simulink subsystem "Plant"  (R2024b)
settings: Solver=VariableStepAuto  StartTime=0.0  StopTime=10.0  RelTol=1e-3
values from neighbouring files (symbols this model uses):
  actuator_delay = 0.1131    [TADPOLEControl.m]
  ipaError = consts(6)    [NonLinearModel.m]
  oxDensityArray = fuelData(1,:)    [MDotODE.m]    (also in oxangle2mdot.m)
  oxError = consts(5)    [NonLinearModel.m]
  oxPressureArray = fuelData(2,:)    [MDotODE.m]    (also in oxangle2mdot.m)
  PcError = consts(7)    [NonLinearModel.m]
undefined symbols (not defined in the file or in its folder): consts, simData, thrustArray
libraries: dspobslib x5
settings Model: Creator=rober  LastModifiedBy=pplat

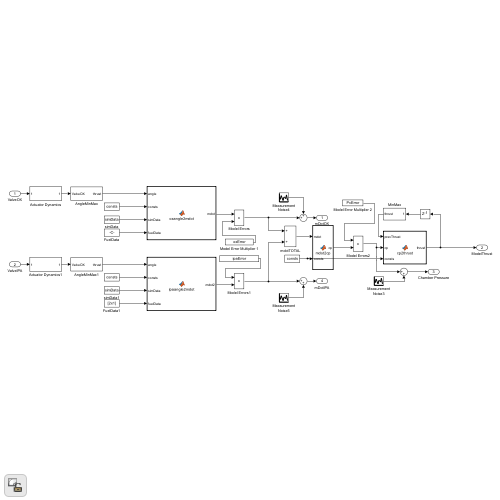
[thumbnail: Simulink's stored preview of the top-level diagram]
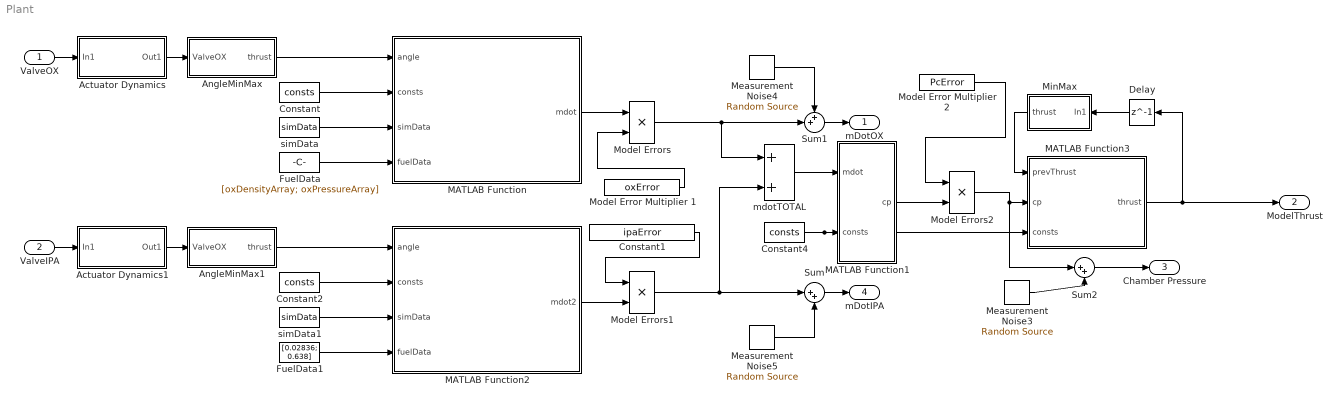
== system Plant ==
  ValveOX : Inport
  ValveIPA : Inport  Port=2
  Actuator Dynamics : Subsystem
  Actuator Dynamics1 : Subsystem
  AngleMinMax : Subsystem
  AngleMinMax1 : Subsystem
  Constant : Constant  Value=consts
  Constant1 : Constant  Value=ipaError
  Constant2 : Constant  Value=consts
  Constant4 : Constant  Value=consts
  Delay : Delay  DelayLength=1  InitialCondition=0  InputProcessing=Columns as channels (frame based)
  FuelData : Constant  Value=[oxDensityArray; oxPressureArray]
  FuelData1 : Constant  Value=[0.02836; 0.638]
  MATLAB Function : MATLAB Function  TreatAsAtomicUnit=on
  MATLAB Function1 : MATLAB Function  TreatAsAtomicUnit=on
  MATLAB Function2 : MATLAB Function  TreatAsAtomicUnit=on
  MATLAB Function3 : MATLAB Function  TreatAsAtomicUnit=on
  Measurement Noise3 : dspobslib/Random Source  SrcType=Gaussian  NormMethod=Ziggurat  CltLength=12  MinVal=0  MaxVal=1  MeanVal=0  VarVal=noise_var_outputs  RepMode=Not repeatable  rawSeed=1  IsInherit=off  SampMode=Continuous  SampTime=1  SampFrame=1  DataType=Double  OutComplex=Real  OutputFrames=off
  Measurement Noise4 : dspobslib/Random Source  SrcType=Gaussian  NormMethod=Ziggurat  CltLength=12  MinVal=0  MaxVal=1  MeanVal=0  VarVal=noise_var_mdot  RepMode=Not repeatable  rawSeed=1  IsInherit=off  SampMode=Continuous  SampTime=1  SampFrame=1  DataType=Double  OutComplex=Real  OutputFrames=off
  Measurement Noise5 : dspobslib/Random Source  SrcType=Gaussian  NormMethod=Ziggurat  CltLength=12  MinVal=0  MaxVal=1  MeanVal=0  VarVal=noise_var_mdot  RepMode=Not repeatable  rawSeed=1  IsInherit=off  SampMode=Continuous  SampTime=1  SampFrame=1  DataType=Double  OutComplex=Real  OutputFrames=off
  MinMax : Subsystem
  Model Error Multiplier 1 : Constant  Value=oxError
  Model Error Multiplier 2 : Constant  Value=PcError
  Model Errors : Product
  Model Errors1 : Product
  Model Errors2 : Product
  Sum : Sum  Inputs=|++
  Sum1 : Sum  Inputs=++|
  Sum2 : Sum  Inputs=|++
  mdotTOTAL : Sum
  simData : Constant  Value=simData
  simData1 : Constant  Value=simData
  mDotOX : Outport
  ModelThrust : Outport  Port=2
  Chamber Pressure : Outport  Port=3
  mDotIPA : Outport  Port=4
  wires:
  Constant/1 -> MATLAB Function/2(consts)
  FuelData/1 -> MATLAB Function/4(fuelData)
  FuelData1/1 -> MATLAB Function2/4(fuelData)
  Constant2/1 -> MATLAB Function2/2(consts)
  Constant4/1 -> MATLAB Function1/2(consts), MATLAB Function3/3(consts)
  mdotTOTAL/1 -> MATLAB Function1/1(mdot)
  Delay/1 -> MinMax/1(In1)
  MinMax/1(thrust) -> MATLAB Function3/1(prevThrust)
  simData/1 -> MATLAB Function/3(simData)
  simData1/1 -> MATLAB Function2/3(simData)
  MATLAB Function3/1(thrust) -> Delay/1, ModelThrust/1
  ValveOX/1 -> Actuator Dynamics/1(In1)
  Actuator Dynamics/1(Out1) -> AngleMinMax/1(ValveOX)
  ValveIPA/1 -> Actuator Dynamics1/1(In1)
  Actuator Dynamics1/1(Out1) -> AngleMinMax1/1(ValveOX)
  Sum/1 -> mDotIPA/1
  Measurement Noise5/1 -> Sum/2
  Sum1/1 -> mDotOX/1
  Measurement Noise3/1 -> Sum2/2
  Sum2/1 -> Chamber Pressure/1
  Model Errors/1 -> mdotTOTAL/1, Sum1/2
  MATLAB Function/1(mdot) -> Model Errors/1
  MATLAB Function2/1(mdot2) -> Model Errors1/2
  Model Errors1/1 -> Sum/1, mdotTOTAL/2
  Model Error Multiplier 1/1 -> Model Errors/2
  AngleMinMax/1(thrust) -> MATLAB Function/1(angle)
  AngleMinMax1/1(thrust) -> MATLAB Function2/1(angle)
  Constant1/1 -> Model Errors1/1
  Model Errors2/1 -> Sum2/1, MATLAB Function3/2(cp)
  MATLAB Function1/1(cp) -> Model Errors2/2
  Model Error Multiplier 2/1 -> Model Errors2/1
  Measurement Noise4/1 -> Sum1/1

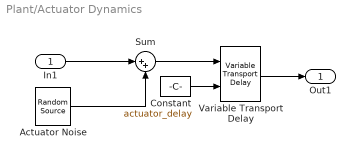
== system Plant/Actuator Dynamics ==
  In1 : Inport
  Actuator Noise : dspobslib/Random Source  SrcType=Gaussian  NormMethod=Ziggurat  CltLength=12  MinVal=0  MaxVal=1  MeanVal=0  VarVal=noise_var_actuators  RepMode=Not repeatable  rawSeed=1  IsInherit=off  SampMode=Continuous  SampTime=1  SampFrame=1  DataType=Double  OutComplex=Real  OutputFrames=off
  Constant : Constant  Value=actuator_delay
  Sum : Sum  Inputs=|++
  Variable Transport Delay : VariableTransportDelay  VariableDelayType=Variable transport delay  MaximumDelay=10  InitialOutput=50  MaximumPoints=2048
  Out1 : Outport
  wires:
  Sum/1 -> Variable Transport Delay/1
  Variable Transport Delay/1 -> Out1/1
  Constant/1 -> Variable Transport Delay/2
  In1/1 -> Sum/1
  Actuator Noise/1 -> Sum/2

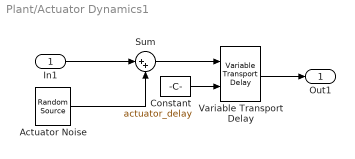
== system Plant/Actuator Dynamics1 ==
  In1 : Inport
  Actuator Noise : dspobslib/Random Source  SrcType=Gaussian  NormMethod=Ziggurat  CltLength=12  MinVal=0  MaxVal=1  MeanVal=0  VarVal=noise_var_actuators  RepMode=Not repeatable  rawSeed=1  IsInherit=off  SampMode=Continuous  SampTime=1  SampFrame=1  DataType=Double  OutComplex=Real  OutputFrames=off
  Constant : Constant  Value=actuator_delay
  Sum : Sum  Inputs=|++
  Variable Transport Delay : VariableTransportDelay  VariableDelayType=Variable transport delay  MaximumDelay=10  InitialOutput=60  MaximumPoints=2048
  Out1 : Outport
  wires:
  Sum/1 -> Variable Transport Delay/1
  Variable Transport Delay/1 -> Out1/1
  Constant/1 -> Variable Transport Delay/2
  In1/1 -> Sum/1
  Actuator Noise/1 -> Sum/2

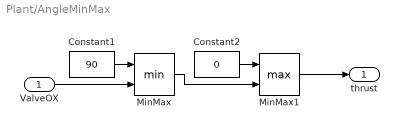
== system Plant/AngleMinMax ==
  ValveOX : Inport
  Constant1 : Constant  Value=90
  Constant2 : Constant  Value=0
  MinMax : MinMax  Inputs=2
  MinMax1 : MinMax  Function=max  Inputs=2
  thrust : Outport
  wires:
  MinMax1/1 -> thrust/1
  ValveOX/1 -> MinMax/2
  MinMax/1 -> MinMax1/2
  Constant1/1 -> MinMax/1
  Constant2/1 -> MinMax1/1

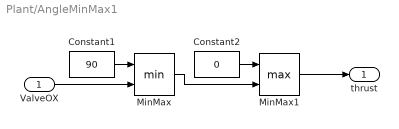
== system Plant/AngleMinMax1 ==
  ValveOX : Inport
  Constant1 : Constant  Value=90
  Constant2 : Constant  Value=0
  MinMax : MinMax  Inputs=2
  MinMax1 : MinMax  Function=max  Inputs=2
  thrust : Outport
  wires:
  MinMax1/1 -> thrust/1
  ValveOX/1 -> MinMax/2
  MinMax/1 -> MinMax1/2
  Constant1/1 -> MinMax/1
  Constant2/1 -> MinMax1/1

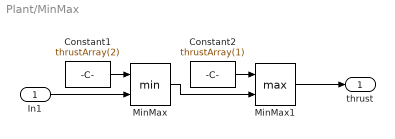
== system Plant/MinMax ==
  In1 : Inport
  Constant1 : Constant  Value=thrustArray(2)
  Constant2 : Constant  Value=thrustArray(1)
  MinMax : MinMax  Inputs=2
  MinMax1 : MinMax  Function=max  Inputs=2
  thrust : Outport
  wires:
  MinMax1/1 -> thrust/1
  In1/1 -> MinMax/2
  MinMax/1 -> MinMax1/2
  Constant1/1 -> MinMax/1
  Constant2/1 -> MinMax1/1

== matlab function Plant/MATLAB Function ==
  data: angle input; mdot output; consts input; simData input; fuelData input
function mdot = oxangle2mdot(angle, consts, simData, fuelData)

    % Conversion Factors and LookUp Arrays
    conversionFactors = [0.004329 60 0.000453592 61023.7];
    subCritVArray = [0.000, 0.070, 0.161, 0.378, 0.670, 1.000, 1.450, 2.050, 2.780, 3.710, 4.960];
    valveAngleArray = [0, 9, 18, 27, 36, 45, 54, 63, 72, 81, 90];
    tempArray = [55, 60, 65, 70, 75, 80, 85, 90, 95, 100, 105, 110, ...
    115, 120, 125, 130, 135, 140, 145, 150];
    oxDensityArray = fuelData(1,:);
    oxPressureArray = fuelData(2,:);

    % cV lookup based off of angle
    subCritV = interp1(valveAngleArray, subCritVArray, angle);

    % ox
    throat = 0.00989;
    cd = 0.975;

    % density and vapour pressure ox
    simData(4);
    density_cv = interp1(tempArray, oxDensityArray, simData(4));
    p_vap = interp1(tempArray, oxPressureArray, simData(4));
    density_valve = interp1(tempArray, oxDensityArray, simData(3));

    %Generates mdot
    alpha = conversionFactors(1)*conversionFactors(2);
    gamma = cd^2*throat^2*2*density_cv*(consts(3)*12);
    beta = conversionFactors(3)*conversionFactors(4);
    deltaP = simData(1)-p_vap;
    mdot = sqrt(subCritV^2*density_valve*(deltaP)*gamma /...
        (alpha^2*gamma*beta + subCritV^2*density_valve));
end

== matlab function Plant/MATLAB Function1 ==
  data: mdot input; cp output; consts input
function cp = mdot2cp(mdot, consts)
    
    cp = mdot*consts(2) / (consts(1)*consts(3));
end

== matlab function Plant/MATLAB Function2 ==
  data: angle input; mdot2 output; consts input; simData input; fuelData input
function mdot2 = ipaangle2mdot(angle, consts, simData, fuelData)

    % Conversion Factors and LookUp Arrays
    conversionFactors = [0.004329 60 0.000453592 61023.7];
    subCritVArray = [0.000, 0.070, 0.161, 0.378, 0.670, 1.000, 1.450, 2.050, 2.780, 3.710, 4.960];
    valveAngleArray = [0, 9, 18, 27, 36, 45, 54, 63, 72, 81, 90];
    tempArray = [55, 60, 65, 70, 75, 80, 85, 90, 95, 100, 105, 110, ...
    115, 120, 125, 130, 135, 140, 145, 150];
    ipaDensityArray = fuelData(1,:);
    ipaPressureArray = fuelData(2,:);

    % cV lookup based off of angle
    subCritV = interp1(valveAngleArray, subCritVArray, angle);

    % ox
    throat = 0.00989;
    cd = 0.975;

    % density and vapour pressure ox
    simData(4);
    density_cv = ipaDensityArray;
    p_vap = ipaPressureArray;
    density_valve = ipaDensityArray;

    %Generates mdot
    alpha = conversionFactors(1)*conversionFactors(2);
    gamma = cd^2*throat^2*2*density_cv*(consts(3)*12);
    beta = conversionFactors(3)*conversionFactors(4);
    deltaP = simData(1)-p_vap;
    mdot2 = sqrt(subCritV^2*density_valve*(deltaP)*gamma /...
        (alpha^2*gamma*beta + subCritV^2*density_valve));
end

== matlab function Plant/MATLAB Function3 ==
  data: prevThrust input; cp input; thrust output; consts input
function thrust = cp2thrust(prevThrust, cp, consts)
  
    thrustArray = [220, 550];
    c_fArray = [1.12, 1.3];
    c_f = interp1(thrustArray, c_fArray, prevThrust);
    thrust = cp*c_f*consts(1);
end
